simulink subsystem "PID_cascade"  (R2024a)
settings: Solver=VariableStepAuto  StartTime=0.0  StopTime=10.0  RelTol=1e-3
undefined symbols (not defined in the file): PID, u_eq
settings Model: Creator=Bocchio  LastModifiedBy=Bocchio

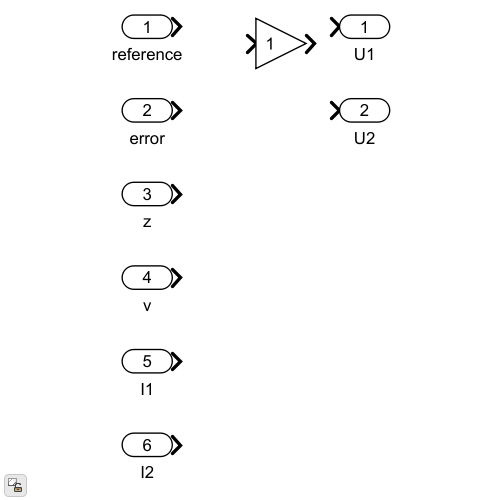
[thumbnail: Simulink's stored preview of the top-level diagram]
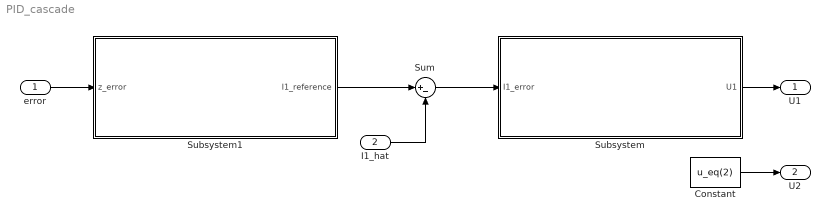
== system PID_cascade ==
  error : Inport
  I1_hat : Inport  Port=2
  Constant : Constant  Value=u_eq(2)
  Subsystem : Subsystem
  Subsystem1 : Subsystem
  Sum : Sum  Inputs=|+-
  U1 : Outport
  U2 : Outport  Port=2
  wires:
  Constant/1 -> U2/1
  I1_hat/1 -> Sum/2
  error/1 -> Subsystem1/1(z_error)
  Subsystem1/1(I1_reference) -> Sum/1
  Sum/1 -> Subsystem/1(I1_error)
  Subsystem/1(U1) -> U1/1

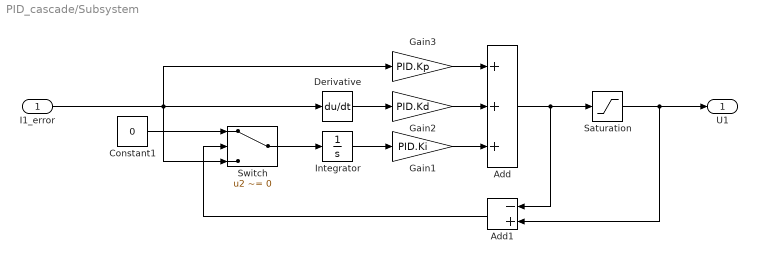
== system PID_cascade/Subsystem ==
  I1_error : Inport
  Add : Sum  Inputs=+++
  Add1 : Sum  Inputs=-+
  Constant1 : Constant  Value=0
  Derivative : Derivative  CoefficientInTFapproximation=1e6
  Gain1 : Gain  Gain=PID.Ki
  Gain2 : Gain  Gain=PID.Kd
  Gain3 : Gain  Gain=PID.Kp
  Integrator : Integrator
  Saturation : Saturate  UpperLimit=1  LowerLimit=0
  Switch : Switch  Criteria=u2 ~= 0  SaturateOnIntegerOverflow=off  InputSameDT=off
  U1 : Outport
  wires:
  Constant1/1 -> Switch/1
  Gain3/1 -> Add/1
  Add1/1 -> Switch/2
  Saturation/1 -> Add1/2, U1/1
  Switch/1 -> Integrator/1
  Add/1 -> Add1/1, Saturation/1
  Integrator/1 -> Gain1/1
  Derivative/1 -> Gain2/1
  Gain1/1 -> Add/3
  Gain2/1 -> Add/2
  I1_error/1 -> Switch/3, Gain3/1, Derivative/1

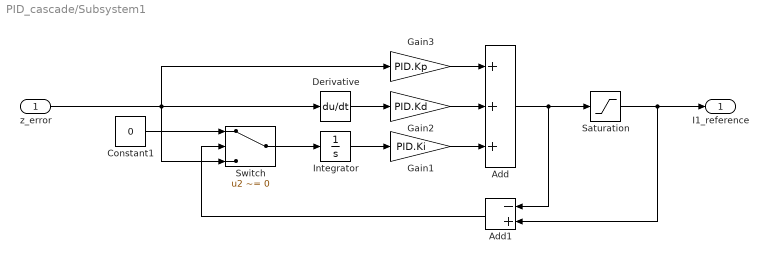
== system PID_cascade/Subsystem1 ==
  z_error : Inport
  Add : Sum  Inputs=+++
  Add1 : Sum  Inputs=-+
  Constant1 : Constant  Value=0
  Derivative : Derivative  CoefficientInTFapproximation=1e6
  Gain1 : Gain  Gain=PID.Ki
  Gain2 : Gain  Gain=PID.Kd
  Gain3 : Gain  Gain=PID.Kp
  Integrator : Integrator
  Saturation : Saturate  UpperLimit=1  LowerLimit=0
  Switch : Switch  Criteria=u2 ~= 0  SaturateOnIntegerOverflow=off  InputSameDT=off
  I1_reference : Outport
  wires:
  z_error/1 -> Derivative/1, Gain3/1, Switch/3
  Gain2/1 -> Add/2
  Gain1/1 -> Add/3
  Derivative/1 -> Gain2/1
  Integrator/1 -> Gain1/1
  Add/1 -> Saturation/1, Add1/1
  Switch/1 -> Integrator/1
  Saturation/1 -> I1_reference/1, Add1/2
  Add1/1 -> Switch/2
  Gain3/1 -> Add/1
  Constant1/1 -> Switch/1
